simulink library "lib_energy_storage2"  (Simulink 10.1)
settings: Solver=VariableStepAuto  StartTime=0.0  StopTime=10.0  RelTol=1e-3
undefined symbols (not defined in the file or in its folder): air_cp, amb_tmp, cyc_mph, enable_stop, ess_cap_scale, ess_cb, ess_cc, ess_coulombic_eff, ess_init_soc, ess_max_ah_cap, ess_max_p, ess_max_p_soc, ess_max_soc, ess_max_volts, ess_min_soc, ess_min_volts, ess_MMi, ess_MMo, ess_mod_airflow, ess_mod_cp, ess_mod_cpm, ess_mod_init_tmp, ess_module_mass, ess_module_num, ess_on, ess_parallel_mod_num, ess_res_scale_coef, ess_res_scale_fun, ess_set_tmp, ess_soc, ess_th_calc, ess_th_res, ess_th_res_off, ess_th_res_on, ess_tmp, ess_voc, fund_byu, fund_byuop, mc_min_volts, saber_air_temp, Saber_Battery_IO_File, saber_init_soc, saber_init_temp, saber_init_voc, saber_k_cb, saber_k_cc, saber_k_rc, saber_k_re, saber_k_rt, saber_k_soc, t_soc, time_step
undefined symbols (not defined in the file): ess_r_chg, ess_r_dis, ess_rc, ess_re, ess_rt, logFlag
libraries: simulink3 x16, lib_energy_storage x1, $bdroot x1
(part 4 of 8)

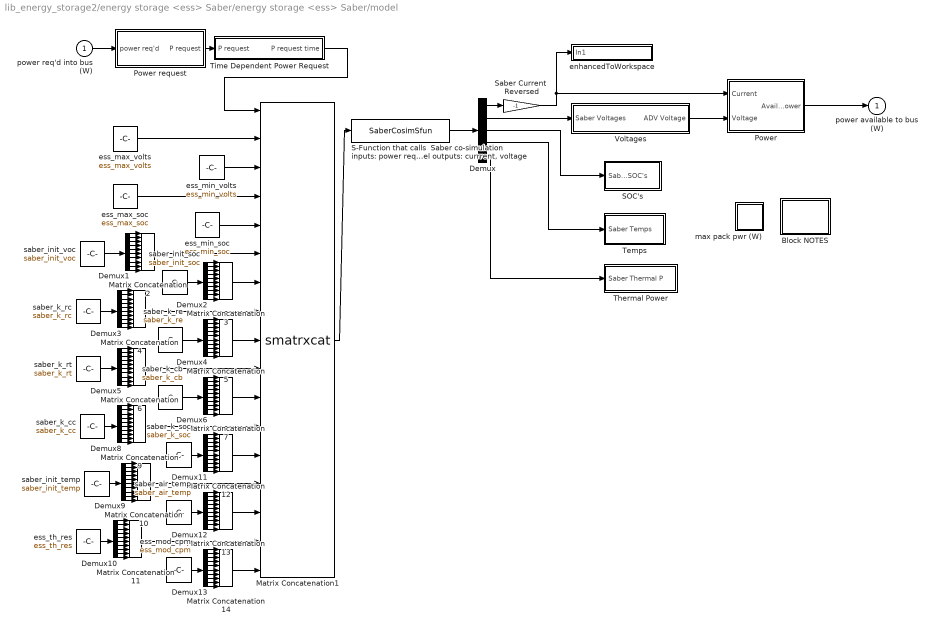
== system lib_energy_storage2/energy storage <ess> Saber/energy storage <ess> Saber/model ==
  power req'd into bus (W) : Inport
  Block NOTES : Subsystem
      mask Display: disp('Block\nNOTES')
  Demux : Demux  Outputs=[1 10 10 10 10]
  Demux{1..6,8..13} (12 alike) : Demux  Outputs=10
  Matrix Concatenation1 : S-Function  FunctionName=smatrxcat  Parameters=numInports,catMethod  SFunctionDeploymentMode=off  EnableBusSupport=off  mask(Matrix Concatenation){numInports=17, catMethod=Horizontal}
      mask prompts: numInports "Number of inputs:"; catMethod "Concatenation method:"
      mask help: Perform horizontal or vertical concatenation. 1-D vector input signals are treated as column vectors, i.e., [Mx1] matrices. The output is always a matrix.
      mask init:
      | xy = matrxcatmask('icon');
      mask TypeOptions catMethod: Horizontal | Vertical
      mask Display:
      | plot(xy.x,xy.y);
      | text(0.15,0.86,xy.label);
  Matrix Concatenation{2..7,9..14} (12 alike) : simulink3/Signals & Systems/Matrix Concatenation  numInports=10  catMethod=Horizontal
      settings: SourceProductBaseCode=SL
  Power : Subsystem
  Power request : Subsystem  AncestorBlock=lib_energy_storage/Ess Choices/energy storage <ess> Saber/Power request
  "S-Function that calls  Saber co-simulation inputs: power request load parameters outputs: accessory power model outputs: currrent, voltage" : S-Function  FunctionName=SaberCosimSfun  Parameters=strrep(which('advisor'),'advisor.m','tmp\'),time_step,Saber_Battery_IO_File  SFunctionDeploymentMode=off  EnableBusSupport=off
  SOC's : Subsystem
  Saber Current  Reversed : Gain  Gain=-1  SaturateOnIntegerOverflow=on
  Temps : Subsystem
  Thermal Power : Subsystem
  Time Dependent Power Request : Subsystem  AncestorBlock=lib_energy_storage/Ess Choices/energy storage <ess> Saber/Time Dependent Power Request
  Voltages : Subsystem
  enhancedToWorkspace : Subsystem  TreatAsAtomicUnit=on  mask(enhancedToWorkspace){generalName=generalName, specificName=current, logFlag=logFlag}
      mask prompts: generalName "General Name [char-evaluated]"; specificName "Specific Name [char-literal]"; logFlag "Enable flag (1=on,0=off)"
      mask help: A wrapper for the Simulink "To Workspace" block that allows you to evaluate the name of the variable to log to workspace. This is useful to avoid the double logging errors that occur when you pull in two library models that attempt to log to the same variable.
      mask init:
      | enhancedToWsMaker
      settings: CopyFcn=breakLinkCopyFcn  ParentCloseFcn=breakLinkParCloseFcn
      mask Help:
      | <h2>Enhanced To Workspace Block</h2>
      | <h3>Parameters</h3>
      | <UL>
      | <li><b>General Name:</b> This is the more general name of the variable. Variables are saved to the workspace as <i>generalName_specificName</i>. Note that this is an evaluated variable. If you would like to type in the value directly, it must be surrounded with single quotes. Otherwise you can input the name of a variable containing a char string.</li>
      | <li><b>Specific Name:</b> This is the specific name of the variable. Note that this is input as a char literal (i.e., you don't need quotes).</li>
      | <li><b>Enable Flag:</b> This flag should have the value of 0 or 1. If 0, the variable will not be logged to the workspace. If 1, the variable will be logged. This is done so that variable logging can be turned off to improve speed.</li>
      | </ul>
      | <h3>Overview</h3>
      | <p>The enhanced to workspace block was put together to allow one to dynamically resolve variable names at run time in simulink. This is most powerful when used in conjunction with a masked subsystem to allow multiple instances of that masked subsytem to be used in the same model. The strategy is to set the generalName in the block mask which will allow the block to change the general name for all variable logging on the fly.
      | <h3>Helper Files</h3>
      | <p>Three m-files are required by the enhancedToWorkspace block. These files are located in the &lt; ADVISOR root &gt;/GUI directory :
      | <ul>
      | <li><i>enhancedToWsMaker.m</i> This file runs the mask initialization for the block</li>
      | <li><i>breakLinkCopyFcn.m</i> This file is used by the block callback when the simulink block is copied. It is necessary to break the link to the enhancedToWorkspace similar to the To Workspace block in order for it to be able to configure itself. (Try copying simulink's To Workspace block--it is impossible to make a link)</li>
      | <li><i>breakLinkParCloseFcn.m</i> This file is similar to the breakLinkCopyFcn and is used when a parent system is closed</li>
      | </ul>
      | <hr>
      | 
      | <p>Created 2003-Jan-21, Michael Patrick O'Keefe, NREL</p>
      | 
      | <!--
      | <VARDEF>
      | <H3>var_name</H3>
      | <UL>
      | <LI><B>data type</B> data type here</LI>
      | <LI><B>units</B> units here</LI>
      | <LI><B>vehicle type</B> vehicle type here</LI>
      | <LI><B>description</B> description here</LI>
      | </UL>
      | </VARDEF>
      | -->
      mask Display: disp([generalName,'_',specificName])
  ess_max_soc : Constant  Value=ess_max_soc
  ess_max_volts : Constant  Value=ess_max_volts
  ess_min_soc : Constant  Value=ess_min_soc
  ess_min_volts : Constant  Value=ess_min_volts
  ess_mod_cpm : Constant  Value=ess_mod_cpm
  ess_th_res : Constant  Value=ess_th_res
  max pack pwr (W) : Subsystem
  saber_air_temp : Constant  Value=saber_air_temp
  saber_init_soc : Constant  Value=saber_init_soc
  saber_init_temp : Constant  Value=saber_init_temp
  saber_init_voc : Constant  Value=saber_init_voc
  saber_k_cb : Constant  Value=saber_k_cb
  saber_k_cc : Constant  Value=saber_k_cc
  saber_k_rc : Constant  Value=saber_k_rc
  saber_k_re : Constant  Value=saber_k_re
  saber_k_rt : Constant  Value=saber_k_rt
  saber_k_soc : Constant  Value=saber_k_soc
  power available to bus (W) : Outport  InitialOutput=0
  wires:
  "S-Function that calls  Saber co-simulation inputs: power request load parameters outputs: accessory power model outputs: currrent, voltage"/1 -> Demux/1
  Demux/2 -> Voltages/1(Saber Voltages)
  Demux/4 -> Temps/1(Saber Temps)
  Demux/3 -> SOC's/1(Saber SOC's)
  Voltages/1(ADV Voltage) -> Power/2(Voltage)
  Power/1(Avail Power) -> power available to bus (W)/1
  Demux/1 -> Saber Current  Reversed/1
  Saber Current  Reversed/1 -> Power/1(Current), enhancedToWorkspace/1(In1)
  Demux/5 -> Thermal Power/1(Saber Thermal P)
  power req'd into bus (W)/1 -> Power request/1(power req'd)
  Matrix Concatenation1/1 -> "S-Function that calls  Saber co-simulation inputs: power request load parameters outputs: accessory power model outputs: currrent, voltage"/1
  Time Dependent Power Request/1(P request time) -> Matrix Concatenation1/1
  ess_max_volts/1 -> Matrix Concatenation1/2
  ess_min_volts/1 -> Matrix Concatenation1/3
  ess_max_soc/1 -> Matrix Concatenation1/4
  ess_min_soc/1 -> Matrix Concatenation1/5
  Demux1/1 -> Matrix Concatenation2/1
  Demux1/2 -> Matrix Concatenation2/2
  Demux1/3 -> Matrix Concatenation2/3
  Demux1/4 -> Matrix Concatenation2/4
  Demux1/5 -> Matrix Concatenation2/5
  Demux1/6 -> Matrix Concatenation2/6
  Demux1/7 -> Matrix Concatenation2/7
  Demux1/8 -> Matrix Concatenation2/8
  Demux1/9 -> Matrix Concatenation2/9
  Demux1/10 -> Matrix Concatenation2/10
  saber_init_soc/1 -> Demux2/1
  Demux2/1 -> Matrix Concatenation3/1
  Demux2/2 -> Matrix Concatenation3/2
  Demux2/3 -> Matrix Concatenation3/3
  Demux2/4 -> Matrix Concatenation3/4
  Demux2/5 -> Matrix Concatenation3/5
  Demux2/6 -> Matrix Concatenation3/6
  Demux2/7 -> Matrix Concatenation3/7
  Demux2/8 -> Matrix Concatenation3/8
  Demux2/9 -> Matrix Concatenation3/9
  Demux2/10 -> Matrix Concatenation3/10
  saber_k_rc/1 -> Demux3/1
  Demux3/1 -> Matrix Concatenation4/1
  Demux3/2 -> Matrix Concatenation4/2
  Demux3/3 -> Matrix Concatenation4/3
  Demux3/4 -> Matrix Concatenation4/4
  Demux3/5 -> Matrix Concatenation4/5
  Demux3/6 -> Matrix Concatenation4/6
  Demux3/7 -> Matrix Concatenation4/7
  Demux3/8 -> Matrix Concatenation4/8
  Demux3/9 -> Matrix Concatenation4/9
  Demux3/10 -> Matrix Concatenation4/10
  saber_k_re/1 -> Demux4/1
  Demux4/1 -> Matrix Concatenation5/1
  Demux4/2 -> Matrix Concatenation5/2
  Demux4/3 -> Matrix Concatenation5/3
  Demux4/4 -> Matrix Concatenation5/4
  Demux4/5 -> Matrix Concatenation5/5
  Demux4/6 -> Matrix Concatenation5/6
  Demux4/7 -> Matrix Concatenation5/7
  Demux4/8 -> Matrix Concatenation5/8
  Demux4/9 -> Matrix Concatenation5/9
  Demux4/10 -> Matrix Concatenation5/10
  Demux5/1 -> Matrix Concatenation6/1
  Demux5/2 -> Matrix Concatenation6/2
  Demux5/3 -> Matrix Concatenation6/3
  Demux5/4 -> Matrix Concatenation6/4
  Demux5/5 -> Matrix Concatenation6/5
  Demux5/6 -> Matrix Concatenation6/6
  Demux5/7 -> Matrix Concatenation6/7
  Demux5/8 -> Matrix Concatenation6/8
  Demux5/9 -> Matrix Concatenation6/9
  Demux5/10 -> Matrix Concatenation6/10
  saber_k_cb/1 -> Demux6/1
  Demux6/1 -> Matrix Concatenation7/1
  Demux6/2 -> Matrix Concatenation7/2
  Demux6/3 -> Matrix Concatenation7/3
  Demux6/4 -> Matrix Concatenation7/4
  Demux6/5 -> Matrix Concatenation7/5
  Demux6/6 -> Matrix Concatenation7/6
  Demux6/7 -> Matrix Concatenation7/7
  Demux6/8 -> Matrix Concatenation7/8
  Demux6/9 -> Matrix Concatenation7/9
  Demux6/10 -> Matrix Concatenation7/10
  saber_k_rt/1 -> Demux5/1
  Matrix Concatenation2/1 -> Matrix Concatenation1/6
  saber_init_voc/1 -> Demux1/1
  Matrix Concatenation3/1 -> Matrix Concatenation1/7
  Matrix Concatenation4/1 -> Matrix Concatenation1/8
  Matrix Concatenation6/1 -> Matrix Concatenation1/10
  Matrix Concatenation7/1 -> Matrix Concatenation1/11
  Matrix Concatenation5/1 -> Matrix Concatenation1/9
  saber_k_cc/1 -> Demux8/1
  Demux8/1 -> Matrix Concatenation9/1
  Demux8/2 -> Matrix Concatenation9/2
  Demux8/3 -> Matrix Concatenation9/3
  Demux8/4 -> Matrix Concatenation9/4
  Demux8/5 -> Matrix Concatenation9/5
  Demux8/6 -> Matrix Concatenation9/6
  Demux8/7 -> Matrix Concatenation9/7
  Demux8/8 -> Matrix Concatenation9/8
  Demux8/9 -> Matrix Concatenation9/9
  Demux8/10 -> Matrix Concatenation9/10
  saber_init_temp/1 -> Demux9/1
  Demux9/1 -> Matrix Concatenation10/1
  Demux9/2 -> Matrix Concatenation10/2
  Demux9/3 -> Matrix Concatenation10/3
  Demux9/4 -> Matrix Concatenation10/4
  Demux9/5 -> Matrix Concatenation10/5
  Demux9/6 -> Matrix Concatenation10/6
  Demux9/7 -> Matrix Concatenation10/7
  Demux9/8 -> Matrix Concatenation10/8
  Demux9/9 -> Matrix Concatenation10/9
  Demux9/10 -> Matrix Concatenation10/10
  ess_th_res/1 -> Demux10/1
  Demux10/1 -> Matrix Concatenation11/1
  Demux10/2 -> Matrix Concatenation11/2
  Demux10/3 -> Matrix Concatenation11/3
  Demux10/4 -> Matrix Concatenation11/4
  Demux10/5 -> Matrix Concatenation11/5
  Demux10/6 -> Matrix Concatenation11/6
  Demux10/7 -> Matrix Concatenation11/7
  Demux10/8 -> Matrix Concatenation11/8
  Demux10/9 -> Matrix Concatenation11/9
  Demux10/10 -> Matrix Concatenation11/10
  saber_k_soc/1 -> Demux11/1
  Demux11/1 -> Matrix Concatenation12/1
  Demux11/2 -> Matrix Concatenation12/2
  Demux11/3 -> Matrix Concatenation12/3
  Demux11/4 -> Matrix Concatenation12/4
  Demux11/5 -> Matrix Concatenation12/5
  Demux11/6 -> Matrix Concatenation12/6
  Demux11/7 -> Matrix Concatenation12/7
  Demux11/8 -> Matrix Concatenation12/8
  Demux11/9 -> Matrix Concatenation12/9
  Demux11/10 -> Matrix Concatenation12/10
  Matrix Concatenation12/1 -> Matrix Concatenation1/13
  saber_air_temp/1 -> Demux12/1
  Demux12/1 -> Matrix Concatenation13/1
  Demux12/2 -> Matrix Concatenation13/2
  Demux12/3 -> Matrix Concatenation13/3
  Demux12/4 -> Matrix Concatenation13/4
  Demux12/5 -> Matrix Concatenation13/5
  Demux12/6 -> Matrix Concatenation13/6
  Demux12/7 -> Matrix Concatenation13/7
  Demux12/8 -> Matrix Concatenation13/8
  Demux12/9 -> Matrix Concatenation13/9
  Demux12/10 -> Matrix Concatenation13/10
  Matrix Concatenation13/1 -> Matrix Concatenation1/15
  ess_mod_cpm/1 -> Demux13/1
  Demux13/1 -> Matrix Concatenation14/1
  Demux13/2 -> Matrix Concatenation14/2
  Demux13/3 -> Matrix Concatenation14/3
  Demux13/4 -> Matrix Concatenation14/4
  Demux13/5 -> Matrix Concatenation14/5
  Demux13/6 -> Matrix Concatenation14/6
  Matrix Concatenation14/1 -> Matrix Concatenation1/17
  Matrix Concatenation9/1 -> Matrix Concatenation1/12
  Matrix Concatenation10/1 -> Matrix Concatenation1/14
  Matrix Concatenation11/1 -> Matrix Concatenation1/16
  Demux13/7 -> Matrix Concatenation14/7
  Demux13/9 -> Matrix Concatenation14/9
  Demux13/8 -> Matrix Concatenation14/8
  Demux13/10 -> Matrix Concatenation14/10
  Power request/1(P request) -> Time Dependent Power Request/1(P request)

== system lib_energy_storage2/energy storage <ess> Saber/energy storage <ess> Saber/signal annotator ==
  In1 : Inport
  Out1 : Outport
  wires:
  In1/1 -> Out1/1  "ess_pwr_out_r"

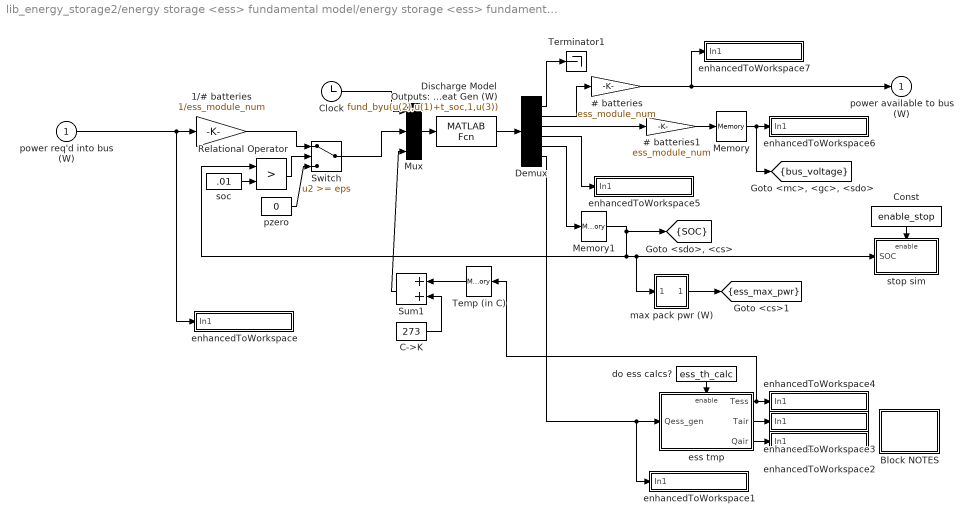
== system lib_energy_storage2/energy storage <ess> fundamental model/energy storage <ess> fundamental model/model ==
  power req'd into bus (W) : Inport
  # batteries : Gain  Gain=ess_module_num  SaturateOnIntegerOverflow=on
  # batteries1 : Gain  Gain=ess_module_num  SaturateOnIntegerOverflow=on
  1/# batteries : Gain  Gain=1/ess_module_num  SaturateOnIntegerOverflow=on
  Block NOTES : Subsystem
      mask Display: disp('Block\nNOTES')
  C->K : Constant  Value=273
  Clock : Clock
  Const : Constant  Value=enable_stop
  Demux : Demux  Outputs=6
  Discharge Model Outputs: Preq(W) Pavail (W) Voltage (V) Current (A) SOC Heat Gen (W) : MATLABFcn  MATLABFcn=fund_byu(u(2),u(1)+t_soc,1,u(3))
  Memory : Memory  InitialCondition=12*ess_module_num
  Memory1 : Memory  InitialCondition=ess_init_soc
  Mux : Mux  Inputs=3
  Relational Operator : RelationalOperator  Operator=>  RndMeth=Nearest  InputSameDT=on
  Sum1 : Sum  SaturateOnIntegerOverflow=on
  Switch : Switch  Threshold=eps  SaturateOnIntegerOverflow=on  InputSameDT=on
  Temp (in C) : Memory  InitialCondition=amb_tmp
  Terminator1 : Terminator
  do ess calcs? : Constant  Value=ess_th_calc
  enhancedToWorkspace : Subsystem  TreatAsAtomicUnit=on  mask(enhancedToWorkspace){generalName=generalName, specificName=pwr_out_r, logFlag=logFlag}
      mask prompts: generalName "General Name [char-evaluated]"; specificName "Specific Name [char-literal]"; logFlag "Enable flag (1=on,0=off)"
      mask help: A wrapper for the Simulink "To Workspace" block that allows you to evaluate the name of the variable to log to workspace. This is useful to avoid the double logging errors that occur when you pull in two library models that attempt to log to the same variable.
      mask init:
      | enhancedToWsMaker
      settings: CopyFcn=breakLinkCopyFcn  ParentCloseFcn=breakLinkParCloseFcn
      mask Help:
      | <h2>Enhanced To Workspace Block</h2>
      | <h3>Parameters</h3>
      | <UL>
      | <li><b>General Name:</b> This is the more general name of the variable. Variables are saved to the workspace as <i>generalName_specificName</i>. Note that this is an evaluated variable. If you would like to type in the value directly, it must be surrounded with single quotes. Otherwise you can input the name of a variable containing a char string.</li>
      | <li><b>Specific Name:</b> This is the specific name of the variable. Note that this is input as a char literal (i.e., you don't need quotes).</li>
      | <li><b>Enable Flag:</b> This flag should have the value of 0 or 1. If 0, the variable will not be logged to the workspace. If 1, the variable will be logged. This is done so that variable logging can be turned off to improve speed.</li>
      | </ul>
      | <h3>Overview</h3>
      | <p>The enhanced to workspace block was put together to allow one to dynamically resolve variable names at run time in simulink. This is most powerful when used in conjunction with a masked subsystem to allow multiple instances of that masked subsytem to be used in the same model. The strategy is to set the generalName in the block mask which will allow the block to change the general name for all variable logging on the fly.
      | <h3>Helper Files</h3>
      | <p>Three m-files are required by the enhancedToWorkspace block. These files are located in the &lt; ADVISOR root &gt;/GUI directory :
      | <ul>
      | <li><i>enhancedToWsMaker.m</i> This file runs the mask initialization for the block</li>
      | <li><i>breakLinkCopyFcn.m</i> This file is used by the block callback when the simulink block is copied. It is necessary to break the link to the enhancedToWorkspace similar to the To Workspace block in order for it to be able to configure itself. (Try copying simulink's To Workspace block--it is impossible to make a link)</li>
      | <li><i>breakLinkParCloseFcn.m</i> This file is similar to the breakLinkCopyFcn and is used when a parent system is closed</li>
      | </ul>
      | <hr>
      | 
      | <p>Created 2003-Jan-21, Michael Patrick O'Keefe, NREL</p>
      | 
      | <!--
      | <VARDEF>
      | <H3>var_name</H3>
      | <UL>
      | <LI><B>data type</B> data type here</LI>
      | <LI><B>units</B> units here</LI>
      | <LI><B>vehicle type</B> vehicle type here</LI>
      | <LI><B>description</B> description here</LI>
      | </UL>
      | </VARDEF>
      | -->
      mask Display: disp([generalName,'_',specificName])
  enhancedToWorkspace1 : Subsystem  TreatAsAtomicUnit=on  mask(enhancedToWorkspace){generalName=generalName, specificName=pwr_loss_a, logFlag=logFlag}
      mask prompts: generalName "General Name [char-evaluated]"; specificName "Specific Name [char-literal]"; logFlag "Enable flag (1=on,0=off)"
      mask help: A wrapper for the Simulink "To Workspace" block that allows you to evaluate the name of the variable to log to workspace. This is useful to avoid the double logging errors that occur when you pull in two library models that attempt to log to the same variable.
      mask init:
      | enhancedToWsMaker
      settings: CopyFcn=breakLinkCopyFcn  ParentCloseFcn=breakLinkParCloseFcn
      mask Help:
      | <h2>Enhanced To Workspace Block</h2>
      | <h3>Parameters</h3>
      | <UL>
      | <li><b>General Name:</b> This is the more general name of the variable. Variables are saved to the workspace as <i>generalName_specificName</i>. Note that this is an evaluated variable. If you would like to type in the value directly, it must be surrounded with single quotes. Otherwise you can input the name of a variable containing a char string.</li>
      | <li><b>Specific Name:</b> This is the specific name of the variable. Note that this is input as a char literal (i.e., you don't need quotes).</li>
      | <li><b>Enable Flag:</b> This flag should have the value of 0 or 1. If 0, the variable will not be logged to the workspace. If 1, the variable will be logged. This is done so that variable logging can be turned off to improve speed.</li>
      | </ul>
      | <h3>Overview</h3>
      | <p>The enhanced to workspace block was put together to allow one to dynamically resolve variable names at run time in simulink. This is most powerful when used in conjunction with a masked subsystem to allow multiple instances of that masked subsytem to be used in the same model. The strategy is to set the generalName in the block mask which will allow the block to change the general name for all variable logging on the fly.
      | <h3>Helper Files</h3>
      | <p>Three m-files are required by the enhancedToWorkspace block. These files are located in the &lt; ADVISOR root &gt;/GUI directory :
      | <ul>
      | <li><i>enhancedToWsMaker.m</i> This file runs the mask initialization for the block</li>
      | <li><i>breakLinkCopyFcn.m</i> This file is used by the block callback when the simulink block is copied. It is necessary to break the link to the enhancedToWorkspace similar to the To Workspace block in order for it to be able to configure itself. (Try copying simulink's To Workspace block--it is impossible to make a link)</li>
      | <li><i>breakLinkParCloseFcn.m</i> This file is similar to the breakLinkCopyFcn and is used when a parent system is closed</li>
      | </ul>
      | <hr>
      | 
      | <p>Created 2003-Jan-21, Michael Patrick O'Keefe, NREL</p>
      | 
      | <!--
      | <VARDEF>
      | <H3>var_name</H3>
      | <UL>
      | <LI><B>data type</B> data type here</LI>
      | <LI><B>units</B> units here</LI>
      | <LI><B>vehicle type</B> vehicle type here</LI>
      | <LI><B>description</B> description here</LI>
      | </UL>
      | </VARDEF>
      | -->
      mask Display: disp([generalName,'_',specificName])
  enhancedToWorkspace2 : Subsystem  TreatAsAtomicUnit=on  mask(enhancedToWorkspace){generalName=generalName, specificName=air_th_pwr, logFlag=logFlag}
      mask prompts: generalName "General Name [char-evaluated]"; specificName "Specific Name [char-literal]"; logFlag "Enable flag (1=on,0=off)"
      mask help: A wrapper for the Simulink "To Workspace" block that allows you to evaluate the name of the variable to log to workspace. This is useful to avoid the double logging errors that occur when you pull in two library models that attempt to log to the same variable.
      mask init:
      | enhancedToWsMaker
      settings: CopyFcn=breakLinkCopyFcn  ParentCloseFcn=breakLinkParCloseFcn
      mask Help:
      | <h2>Enhanced To Workspace Block</h2>
      | <h3>Parameters</h3>
      | <UL>
      | <li><b>General Name:</b> This is the more general name of the variable. Variables are saved to the workspace as <i>generalName_specificName</i>. Note that this is an evaluated variable. If you would like to type in the value directly, it must be surrounded with single quotes. Otherwise you can input the name of a variable containing a char string.</li>
      | <li><b>Specific Name:</b> This is the specific name of the variable. Note that this is input as a char literal (i.e., you don't need quotes).</li>
      | <li><b>Enable Flag:</b> This flag should have the value of 0 or 1. If 0, the variable will not be logged to the workspace. If 1, the variable will be logged. This is done so that variable logging can be turned off to improve speed.</li>
      | </ul>
      | <h3>Overview</h3>
      | <p>The enhanced to workspace block was put together to allow one to dynamically resolve variable names at run time in simulink. This is most powerful when used in conjunction with a masked subsystem to allow multiple instances of that masked subsytem to be used in the same model. The strategy is to set the generalName in the block mask which will allow the block to change the general name for all variable logging on the fly.
      | <h3>Helper Files</h3>
      | <p>Three m-files are required by the enhancedToWorkspace block. These files are located in the &lt; ADVISOR root &gt;/GUI directory :
      | <ul>
      | <li><i>enhancedToWsMaker.m</i> This file runs the mask initialization for the block</li>
      | <li><i>breakLinkCopyFcn.m</i> This file is used by the block callback when the simulink block is copied. It is necessary to break the link to the enhancedToWorkspace similar to the To Workspace block in order for it to be able to configure itself. (Try copying simulink's To Workspace block--it is impossible to make a link)</li>
      | <li><i>breakLinkParCloseFcn.m</i> This file is similar to the breakLinkCopyFcn and is used when a parent system is closed</li>
      | </ul>
      | <hr>
      | 
      | <p>Created 2003-Jan-21, Michael Patrick O'Keefe, NREL</p>
      | 
      | <!--
      | <VARDEF>
      | <H3>var_name</H3>
      | <UL>
      | <LI><B>data type</B> data type here</LI>
      | <LI><B>units</B> units here</LI>
      | <LI><B>vehicle type</B> vehicle type here</LI>
      | <LI><B>description</B> description here</LI>
      | </UL>
      | </VARDEF>
      | -->
      mask Display: disp([generalName,'_',specificName])
  enhancedToWorkspace3 : Subsystem  TreatAsAtomicUnit=on  mask(enhancedToWorkspace){generalName=generalName, specificName=air_tmp, logFlag=logFlag}
      mask prompts: generalName "General Name [char-evaluated]"; specificName "Specific Name [char-literal]"; logFlag "Enable flag (1=on,0=off)"
      mask help: A wrapper for the Simulink "To Workspace" block that allows you to evaluate the name of the variable to log to workspace. This is useful to avoid the double logging errors that occur when you pull in two library models that attempt to log to the same variable.
      mask init:
      | enhancedToWsMaker
      settings: CopyFcn=breakLinkCopyFcn  ParentCloseFcn=breakLinkParCloseFcn
      mask Help:
      | <h2>Enhanced To Workspace Block</h2>
      | <h3>Parameters</h3>
      | <UL>
      | <li><b>General Name:</b> This is the more general name of the variable. Variables are saved to the workspace as <i>generalName_specificName</i>. Note that this is an evaluated variable. If you would like to type in the value directly, it must be surrounded with single quotes. Otherwise you can input the name of a variable containing a char string.</li>
      | <li><b>Specific Name:</b> This is the specific name of the variable. Note that this is input as a char literal (i.e., you don't need quotes).</li>
      | <li><b>Enable Flag:</b> This flag should have the value of 0 or 1. If 0, the variable will not be logged to the workspace. If 1, the variable will be logged. This is done so that variable logging can be turned off to improve speed.</li>
      | </ul>
      | <h3>Overview</h3>
      | <p>The enhanced to workspace block was put together to allow one to dynamically resolve variable names at run time in simulink. This is most powerful when used in conjunction with a masked subsystem to allow multiple instances of that masked subsytem to be used in the same model. The strategy is to set the generalName in the block mask which will allow the block to change the general name for all variable logging on the fly.
      | <h3>Helper Files</h3>
      | <p>Three m-files are required by the enhancedToWorkspace block. These files are located in the &lt; ADVISOR root &gt;/GUI directory :
      | <ul>
      | <li><i>enhancedToWsMaker.m</i> This file runs the mask initialization for the block</li>
      | <li><i>breakLinkCopyFcn.m</i> This file is used by the block callback when the simulink block is copied. It is necessary to break the link to the enhancedToWorkspace similar to the To Workspace block in order for it to be able to configure itself. (Try copying simulink's To Workspace block--it is impossible to make a link)</li>
      | <li><i>breakLinkParCloseFcn.m</i> This file is similar to the breakLinkCopyFcn and is used when a parent system is closed</li>
      | </ul>
      | <hr>
      | 
      | <p>Created 2003-Jan-21, Michael Patrick O'Keefe, NREL</p>
      | 
      | <!--
      | <VARDEF>
      | <H3>var_name</H3>
      | <UL>
      | <LI><B>data type</B> data type here</LI>
      | <LI><B>units</B> units here</LI>
      | <LI><B>vehicle type</B> vehicle type here</LI>
      | <LI><B>description</B> description here</LI>
      | </UL>
      | </VARDEF>
      | -->
      mask Display: disp([generalName,'_',specificName])
  enhancedToWorkspace4 : Subsystem  TreatAsAtomicUnit=on  mask(enhancedToWorkspace){generalName=generalName, specificName=mod_tmp, logFlag=logFlag}
      mask prompts: generalName "General Name [char-evaluated]"; specificName "Specific Name [char-literal]"; logFlag "Enable flag (1=on,0=off)"
      mask help: A wrapper for the Simulink "To Workspace" block that allows you to evaluate the name of the variable to log to workspace. This is useful to avoid the double logging errors that occur when you pull in two library models that attempt to log to the same variable.
      mask init:
      | enhancedToWsMaker
      settings: CopyFcn=breakLinkCopyFcn  ParentCloseFcn=breakLinkParCloseFcn
      mask Help:
      | <h2>Enhanced To Workspace Block</h2>
      | <h3>Parameters</h3>
      | <UL>
      | <li><b>General Name:</b> This is the more general name of the variable. Variables are saved to the workspace as <i>generalName_specificName</i>. Note that this is an evaluated variable. If you would like to type in the value directly, it must be surrounded with single quotes. Otherwise you can input the name of a variable containing a char string.</li>
      | <li><b>Specific Name:</b> This is the specific name of the variable. Note that this is input as a char literal (i.e., you don't need quotes).</li>
      | <li><b>Enable Flag:</b> This flag should have the value of 0 or 1. If 0, the variable will not be logged to the workspace. If 1, the variable will be logged. This is done so that variable logging can be turned off to improve speed.</li>
      | </ul>
      | <h3>Overview</h3>
      | <p>The enhanced to workspace block was put together to allow one to dynamically resolve variable names at run time in simulink. This is most powerful when used in conjunction with a masked subsystem to allow multiple instances of that masked subsytem to be used in the same model. The strategy is to set the generalName in the block mask which will allow the block to change the general name for all variable logging on the fly.
      | <h3>Helper Files</h3>
      | <p>Three m-files are required by the enhancedToWorkspace block. These files are located in the &lt; ADVISOR root &gt;/GUI directory :
      | <ul>
      | <li><i>enhancedToWsMaker.m</i> This file runs the mask initialization for the block</li>
      | <li><i>breakLinkCopyFcn.m</i> This file is used by the block callback when the simulink block is copied. It is necessary to break the link to the enhancedToWorkspace similar to the To Workspace block in order for it to be able to configure itself. (Try copying simulink's To Workspace block--it is impossible to make a link)</li>
      | <li><i>breakLinkParCloseFcn.m</i> This file is similar to the breakLinkCopyFcn and is used when a parent system is closed</li>
      | </ul>
      | <hr>
      | 
      | <p>Created 2003-Jan-21, Michael Patrick O'Keefe, NREL</p>
      | 
      | <!--
      | <VARDEF>
      | <H3>var_name</H3>
      | <UL>
      | <LI><B>data type</B> data type here</LI>
      | <LI><B>units</B> units here</LI>
      | <LI><B>vehicle type</B> vehicle type here</LI>
      | <LI><B>description</B> description here</LI>
      | </UL>
      | </VARDEF>
      | -->
      mask Display: disp([generalName,'_',specificName])
  enhancedToWorkspace5 : Subsystem  TreatAsAtomicUnit=on  mask(enhancedToWorkspace){generalName=generalName, specificName=current, logFlag=logFlag}
      mask prompts: generalName "General Name [char-evaluated]"; specificName "Specific Name [char-literal]"; logFlag "Enable flag (1=on,0=off)"
      mask help: A wrapper for the Simulink "To Workspace" block that allows you to evaluate the name of the variable to log to workspace. This is useful to avoid the double logging errors that occur when you pull in two library models that attempt to log to the same variable.
      mask init:
      | enhancedToWsMaker
      settings: CopyFcn=breakLinkCopyFcn  ParentCloseFcn=breakLinkParCloseFcn
      mask Help:
      | <h2>Enhanced To Workspace Block</h2>
      | <h3>Parameters</h3>
      | <UL>
      | <li><b>General Name:</b> This is the more general name of the variable. Variables are saved to the workspace as <i>generalName_specificName</i>. Note that this is an evaluated variable. If you would like to type in the value directly, it must be surrounded with single quotes. Otherwise you can input the name of a variable containing a char string.</li>
      | <li><b>Specific Name:</b> This is the specific name of the variable. Note that this is input as a char literal (i.e., you don't need quotes).</li>
      | <li><b>Enable Flag:</b> This flag should have the value of 0 or 1. If 0, the variable will not be logged to the workspace. If 1, the variable will be logged. This is done so that variable logging can be turned off to improve speed.</li>
      | </ul>
      | <h3>Overview</h3>
      | <p>The enhanced to workspace block was put together to allow one to dynamically resolve variable names at run time in simulink. This is most powerful when used in conjunction with a masked subsystem to allow multiple instances of that masked subsytem to be used in the same model. The strategy is to set the generalName in the block mask which will allow the block to change the general name for all variable logging on the fly.
      | <h3>Helper Files</h3>
      | <p>Three m-files are required by the enhancedToWorkspace block. These files are located in the &lt; ADVISOR root &gt;/GUI directory :
      | <ul>
      | <li><i>enhancedToWsMaker.m</i> This file runs the mask initialization for the block</li>
      | <li><i>breakLinkCopyFcn.m</i> This file is used by the block callback when the simulink block is copied. It is necessary to break the link to the enhancedToWorkspace similar to the To Workspace block in order for it to be able to configure itself. (Try copying simulink's To Workspace block--it is impossible to make a link)</li>
      | <li><i>breakLinkParCloseFcn.m</i> This file is similar to the breakLinkCopyFcn and is used when a parent system is closed</li>
      | </ul>
      | <hr>
      | 
      | <p>Created 2003-Jan-21, Michael Patrick O'Keefe, NREL</p>
      | 
      | <!--
      | <VARDEF>
      | <H3>var_name</H3>
      | <UL>
      | <LI><B>data type</B> data type here</LI>
      | <LI><B>units</B> units here</LI>
      | <LI><B>vehicle type</B> vehicle type here</LI>
      | <LI><B>description</B> description here</LI>
      | </UL>
      | </VARDEF>
      | -->
      mask Display: disp([generalName,'_',specificName])
  enhancedToWorkspace6 : Subsystem  TreatAsAtomicUnit=on  mask(enhancedToWorkspace){generalName=generalName, specificName=voltage, logFlag=logFlag}
      mask prompts: generalName "General Name [char-evaluated]"; specificName "Specific Name [char-literal]"; logFlag "Enable flag (1=on,0=off)"
      mask help: A wrapper for the Simulink "To Workspace" block that allows you to evaluate the name of the variable to log to workspace. This is useful to avoid the double logging errors that occur when you pull in two library models that attempt to log to the same variable.
      mask init:
      | enhancedToWsMaker
      settings: CopyFcn=breakLinkCopyFcn  ParentCloseFcn=breakLinkParCloseFcn
      mask Help:
      | <h2>Enhanced To Workspace Block</h2>
      | <h3>Parameters</h3>
      | <UL>
      | <li><b>General Name:</b> This is the more general name of the variable. Variables are saved to the workspace as <i>generalName_specificName</i>. Note that this is an evaluated variable. If you would like to type in the value directly, it must be surrounded with single quotes. Otherwise you can input the name of a variable containing a char string.</li>
      | <li><b>Specific Name:</b> This is the specific name of the variable. Note that this is input as a char literal (i.e., you don't need quotes).</li>
      | <li><b>Enable Flag:</b> This flag should have the value of 0 or 1. If 0, the variable will not be logged to the workspace. If 1, the variable will be logged. This is done so that variable logging can be turned off to improve speed.</li>
      | </ul>
      | <h3>Overview</h3>
      | <p>The enhanced to workspace block was put together to allow one to dynamically resolve variable names at run time in simulink. This is most powerful when used in conjunction with a masked subsystem to allow multiple instances of that masked subsytem to be used in the same model. The strategy is to set the generalName in the block mask which will allow the block to change the general name for all variable logging on the fly.
      | <h3>Helper Files</h3>
      | <p>Three m-files are required by the enhancedToWorkspace block. These files are located in the &lt; ADVISOR root &gt;/GUI directory :
      | <ul>
      | <li><i>enhancedToWsMaker.m</i> This file runs the mask initialization for the block</li>
      | <li><i>breakLinkCopyFcn.m</i> This file is used by the block callback when the simulink block is copied. It is necessary to break the link to the enhancedToWorkspace similar to the To Workspace block in order for it to be able to configure itself. (Try copying simulink's To Workspace block--it is impossible to make a link)</li>
      | <li><i>breakLinkParCloseFcn.m</i> This file is similar to the breakLinkCopyFcn and is used when a parent system is closed</li>
      | </ul>
      | <hr>
      | 
      | <p>Created 2003-Jan-21, Michael Patrick O'Keefe, NREL</p>
      | 
      | <!--
      | <VARDEF>
      | <H3>var_name</H3>
      | <UL>
      | <LI><B>data type</B> data type here</LI>
      | <LI><B>units</B> units here</LI>
      | <LI><B>vehicle type</B> vehicle type here</LI>
      | <LI><B>description</B> description here</LI>
      | </UL>
      | </VARDEF>
      | -->
      mask Display: disp([generalName,'_',specificName])
  enhancedToWorkspace7 : Subsystem  TreatAsAtomicUnit=on  mask(enhancedToWorkspace){generalName=generalName, specificName=pwr_out_a, logFlag=logFlag}
      mask prompts: generalName "General Name [char-evaluated]"; specificName "Specific Name [char-literal]"; logFlag "Enable flag (1=on,0=off)"
      mask help: A wrapper for the Simulink "To Workspace" block that allows you to evaluate the name of the variable to log to workspace. This is useful to avoid the double logging errors that occur when you pull in two library models that attempt to log to the same variable.
      mask init:
      | enhancedToWsMaker
      settings: CopyFcn=breakLinkCopyFcn  ParentCloseFcn=breakLinkParCloseFcn
      mask Help:
      | <h2>Enhanced To Workspace Block</h2>
      | <h3>Parameters</h3>
      | <UL>
      | <li><b>General Name:</b> This is the more general name of the variable. Variables are saved to the workspace as <i>generalName_specificName</i>. Note that this is an evaluated variable. If you would like to type in the value directly, it must be surrounded with single quotes. Otherwise you can input the name of a variable containing a char string.</li>
      | <li><b>Specific Name:</b> This is the specific name of the variable. Note that this is input as a char literal (i.e., you don't need quotes).</li>
      | <li><b>Enable Flag:</b> This flag should have the value of 0 or 1. If 0, the variable will not be logged to the workspace. If 1, the variable will be logged. This is done so that variable logging can be turned off to improve speed.</li>
      | </ul>
      | <h3>Overview</h3>
      | <p>The enhanced to workspace block was put together to allow one to dynamically resolve variable names at run time in simulink. This is most powerful when used in conjunction with a masked subsystem to allow multiple instances of that masked subsytem to be used in the same model. The strategy is to set the generalName in the block mask which will allow the block to change the general name for all variable logging on the fly.
      | <h3>Helper Files</h3>
      | <p>Three m-files are required by the enhancedToWorkspace block. These files are located in the &lt; ADVISOR root &gt;/GUI directory :
      | <ul>
      | <li><i>enhancedToWsMaker.m</i> This file runs the mask initialization for the block</li>
      | <li><i>breakLinkCopyFcn.m</i> This file is used by the block callback when the simulink block is copied. It is necessary to break the link to the enhancedToWorkspace similar to the To Workspace block in order for it to be able to configure itself. (Try copying simulink's To Workspace block--it is impossible to make a link)</li>
      | <li><i>breakLinkParCloseFcn.m</i> This file is similar to the breakLinkCopyFcn and is used when a parent system is closed</li>
      | </ul>
      | <hr>
      | 
      | <p>Created 2003-Jan-21, Michael Patrick O'Keefe, NREL</p>
      | 
      | <!--
      | <VARDEF>
      | <H3>var_name</H3>
      | <UL>
      | <LI><B>data type</B> data type here</LI>
      | <LI><B>units</B> units here</LI>
      | <LI><B>vehicle type</B> vehicle type here</LI>
      | <LI><B>description</B> description here</LI>
      | </UL>
      | </VARDEF>
      | -->
      mask Display: disp([generalName,'_',specificName])
  ess tmp : Subsystem  TreatAsAtomicUnit=on
  max pack pwr (W) : Subsystem
  pzero : Constant  Value=0
  soc : Constant  Value=.01
  stop sim : Subsystem  TreatAsAtomicUnit=on
  power available to bus (W) : Outport  InitialOutput=0
  tag scope: SOC=scoped, bus_voltage=scoped, ess_max_pwr=scoped
  wires:
  ess tmp/1(Tess) -> Temp (in C)/1, enhancedToWorkspace4/1(In1)
  ess tmp/3(Qair) -> enhancedToWorkspace2/1(In1)
  ess tmp/2(Tair) -> enhancedToWorkspace3/1(In1)
  do ess calcs?/1 -> ess tmp/Enable
  Demux/6 -> ess tmp/1(Qess_gen), enhancedToWorkspace1/1(In1)
  max pack pwr (W)/1(ess discharge pwr) -> [ess_max_pwr]
  Const/1 -> stop sim/Enable
  Sum1/1 -> Mux/3
  C->K/1 -> Sum1/2
  Temp (in C)/1 -> Sum1/1
  Memory1/1 -> [SOC], max pack pwr (W)/1(SOC), stop sim/1(SOC), Relational Operator/1
  Memory/1 -> [bus_voltage], enhancedToWorkspace6/1(In1)
  Demux/3 -> # batteries1/1
  # batteries1/1 -> Memory/1
  # batteries/1 -> power available to bus (W)/1, enhancedToWorkspace7/1(In1)
  Demux/1 -> Terminator1/1
  Switch/1 -> Mux/2
  1/# batteries/1 -> Switch/1
  soc/1 -> Relational Operator/2
  Relational Operator/1 -> Switch/2
  pzero/1 -> Switch/3
  power req'd into bus (W)/1 -> 1/# batteries/1, enhancedToWorkspace/1(In1)
  Clock/1 -> Mux/1
  Demux/2 -> # batteries/1
  Demux/4 -> enhancedToWorkspace5/1(In1)
  Demux/5 -> Memory1/1
  Discharge Model Outputs: Preq(W) Pavail (W) Voltage (V) Current (A) SOC Heat Gen (W)/1 -> Demux/1
  Mux/1 -> Discharge Model Outputs: Preq(W) Pavail (W) Voltage (V) Current (A) SOC Heat Gen (W)/1

== system lib_energy_storage2/energy storage <ess> fundamental model/energy storage <ess> fundamental model/signal annotator ==
  In1 : Inport
  Out1 : Outport
  wires:
  In1/1 -> Out1/1  "ess_pwr_out_r"
